simulink model "nonlinearSimMPC"  (R2016a)
settings: Solver=ode45  StartTime=0.0  StopTime=100  FixedStep=1e-3  MaxStep=1e-3  RelTol=1e-3
values from neighbouring files (symbols this model uses):
  x0 = [0 0 0 0]'    [simFullOrderModel.m]    (also in simReducedOrderController.m = H*x0)
libraries: simulink x2
settings Model: Creator=xingye  LastModifiedBy=xingye

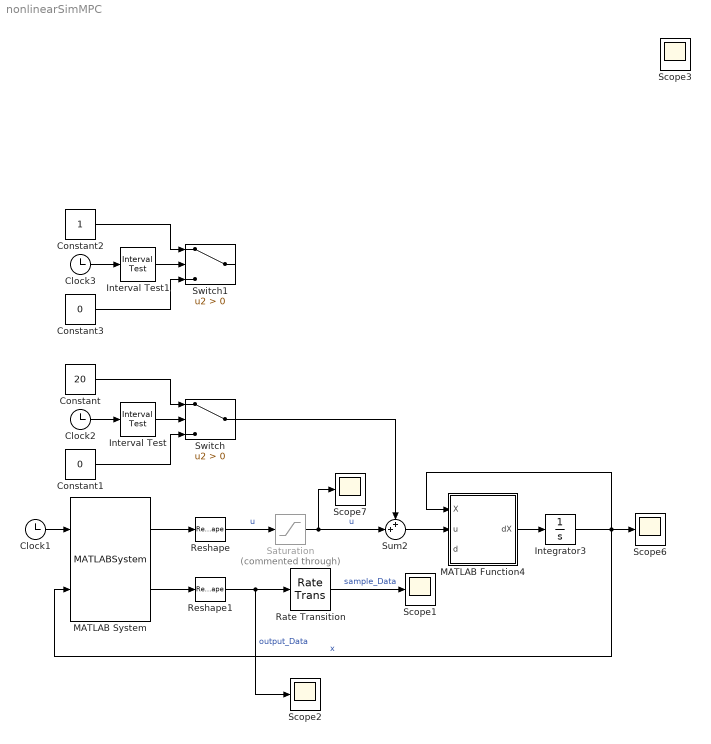
== system nonlinearSimMPC ==
  Clock1 : Clock
  Clock2 : Clock
  Clock3 : Clock
  Constant : Constant  Value=20
  Constant1 : Constant  Value=0
  Constant2 : Constant
  Constant3 : Constant  Value=0
  Integrator3 : Integrator  InitialCondition=x0
  Interval Test : simulink/Logic and Bit Operations/Interval Test  IntervalClosedRight=on  uplimit=70  IntervalClosedLeft=on  lowlimit=69.5  OutDataTypeStr=boolean
  Interval Test1 : simulink/Logic and Bit Operations/Interval Test  IntervalClosedRight=on  uplimit=12  IntervalClosedLeft=on  lowlimit=11.5  OutDataTypeStr=boolean
  MATLAB Function4 : MATLAB Function  TreatAsAtomicUnit=on
  MATLAB System : MATLABSystem  System=ClassControllerEquiState  Taction=Taction  SimulateUsing=Code generation
      mask Type: ClassControllerEquiState
      mask Display:
      | disp('ClassControllerEquiState');
      | port_label('input',1,'t');
      | port_label('input',2,'x');
      | port_label('output',1,'u');
      | port_label('output',2,'output_Data');
  Rate Transition : RateTransition  OutPortSampleTime=2
  Reshape : Reshape
  Reshape1 : Reshape
  Saturation : Saturate  Commented=through  UpperLimit=30  LowerLimit=-30
  Scope{1..3,6..7} (5 alike) : Scope
  Sum2 : Sum  Inputs=++|
  Switch : Switch  Criteria=u2 > Threshold
  Switch1 : Switch  Criteria=u2 > Threshold
  wires:
  MATLAB Function4/1(dX) -> Integrator3/1
  Integrator3/1 -> MATLAB Function4/1(X), Scope6/1, MATLAB System/2  "x"
  Saturation/1 -> Scope7/1, Sum2/2  "u"
  Clock1/1 -> MATLAB System/1
  Rate Transition/1 -> Scope1/1  "sample_Data"
  Constant/1 -> Switch/1
  Switch/1 -> Sum2/1
  Interval Test/1 -> Switch/2
  Clock2/1 -> Interval Test/1
  Constant1/1 -> Switch/3
  Sum2/1 -> MATLAB Function4/2(u)
  Reshape/1 -> Saturation/1  "u"
  MATLAB System/2 -> Reshape1/1
  Constant2/1 -> Switch1/1
  Interval Test1/1 -> Switch1/2
  Clock3/1 -> Interval Test1/1
  Constant3/1 -> Switch1/3
  MATLAB System/1 -> Reshape/1
  Reshape1/1 -> Scope2/1, Rate Transition/1  "output_Data"

== matlab function nonlinearSimMPC/MATLAB Function4 ==
  data: X input; u input; dX output; d input
function dX = fcn(X, u, d)
%#codegen

% X = [0 pi/2 0 0]';
% u = 0;
%%
x = X(1:2);
x(2) = x(2) + pi/2;
xdot = X(3:4);

M = ([[2,-sin(x(2,:))/2];[-sin(x(2,:))/2,1/3]]);
f = ([[u(:,1)-xdot(1,:)/10+(xdot(2,:)^2*cos(x(2,:)))/2];[-xdot(2,:)/100-(981*cos(x(2,:)))/200]]);

f(2) = f(2) + d;
xddot = M\f;

dX = [xdot; xddot];


% y = u;
